simulink model "PMSM_DPCC_NLESO_MRAS"  (R2022a)
settings: Solver=FixedStepDiscrete  StartTime=0.0  StopTime=2  FixedStep=Ts  RelTol=1e-3
InitFcn:
  | Ts = 5e-7;%仿真步长
  | Tpwm = 1e-4;%开关周期
  | Tsample = Tpwm/1;%采样周期/控制周期
  | Tspeed = Tsample;%转速采样周期
  | Pn = 4;%电机极对数
  | Ls = 8.5e-3;%定子电感，采用隐极的，Ld=Lq=Ls
  | Rs = 3;%定子电阻
  | flux = 0.1688;%永磁体磁链
  | Vdc = 311;%直流母线电压
  | iqmax = 20;%额定电流
  | J = 5e-3;%转动惯量
  | B = 2.5e-3;%阻尼系数
  | n_init = 0;%初始转速
  | 
  | %这是DSP内部的控制器参数
  | Ls1 = 1*Ls;%电感参数设置为实际电感
  | Ld1 = Ls1;
  | Lq1 = Ls1;
  | Rs1 = 1*Rs;%电阻参数设置为实际电阻
  | flux1 =1*flux;%磁链参数设置为实际磁链
undefined symbols (not defined in the file): DiscIntNeverNeededParam, magnitude
libraries: simulink x9, slpidlib x2, spsDCVoltageSourceLib x1, spsPermanentMagnetSynchronousMachineLib x1, spsUniversalBridgeLib x1, spspowerguiLib x1
(part 2 of 2)

== matlab function PMSM_DPCC_NLESO_MRAS/SVPWM/电压采集模块 ==
  data: T1 input; udk output; T2 input; N input; uqk output; theta input; Tpwm input; Vdc input; wk input
function [udk,uqk] = fcn(T1,T2,N,theta,Tpwm,Vdc,wk)
%初始化
    Sa1 = 1;
    Sb1 = 1;
    Sc1 = 1;
    
    Sa2 = 1;
    Sb2 = 1;
    Sc2 = 1;
%%
%各个扇区对应的N分布为3 1 5 4 6 2 
%第I扇区的T1对应电压矢量100，T2对应电压矢量110；
%第II扇区的T1对应电压矢量010，T2对应电压矢量110；
%第III扇区的T1对应电压矢量010，T2对应电压矢量011；
%第IV扇区的T1对应电压矢量001，T2对应电压矢量011；
%第V扇区的T1对应电压矢量001，T2对应电压矢量101；
%第VI扇区的T1对应电压矢量100，T2对应电压矢量101；
%%
%翻译一下
%N=1的T1对应电压矢量010，T2对应电压矢量110；
%N=2的T1对应电压矢量100，T2对应电压矢量101；
%N=3的T1对应电压矢量100，T2对应电压矢量110；
%N=4的T1对应电压矢量001，T2对应电压矢量011；
%N=5的T1对应电压矢量010，T2对应电压矢量011；
%N=6的T1对应电压矢量001，T2对应电压矢量101；
%%
%相电压与开关函数的关系为：
%VaN = Vdc/3*(2*Sa-Sb-Sc);
%VbN = Vdc/3*(2*Sb-Sa-Sc);
%VcN = Vdc/3*(2*Sc-Sa-Sb);

if N==1
    Sa1 = 0;
    Sb1 = 1;
    Sc1 = 0;
    
    Sa2 = 1;
    Sb2 = 1;
    Sc2 = 0;
    
    
elseif N==2
    Sa1 = 1;
    Sb1 = 0;
    Sc1 = 0;
    
    Sa2 = 1;
    Sb2 = 0;
    Sc2 = 1;
    
    
 elseif N==3
    Sa1 = 1;
    Sb1 = 0;
    Sc1 = 0;
    
    Sa2 = 1;
    Sb2 = 1;
    Sc2 = 0;
    
    
 elseif N==4
    Sa1 = 0;
    Sb1 = 0;
    Sc1 = 1;
    
    Sa2 = 0;
    Sb2 = 1;
    Sc2 = 1;
    
    
 elseif N==5
    Sa1 = 0;
    Sb1 = 1;
    Sc1 = 0;
    
    Sa2 = 0;
    Sb2 = 1;
    Sc2 = 1;
    
    
 elseif N==6
    Sa1 = 0;
    Sb1 = 0;
    Sc1 = 1;
    
    Sa2 = 1;
    Sb2 = 0;
    Sc2 = 1;
end

VaN = Vdc/3*(2*Sa1-Sb1-Sc1)*T1/Tpwm+Vdc/3*(2*Sa2-Sb2-Sc2)*T2/Tpwm;
VbN = Vdc/3*(2*Sb1-Sa1-Sc1)*T1/Tpwm+Vdc/3*(2*Sb2-Sa2-Sc2)*T2/Tpwm;
VcN = Vdc/3*(2*Sc1-Sa1-Sb1)*T1/Tpwm+Vdc/3*(2*Sc2-Sa2-Sb2)*T2/Tpwm;

    
    if wk==0
        m = 1;
    else
        m = (2*sin(0.5*wk*Tpwm))/(wk*Tpwm);%平均值系数
    end
	theta_compen = theta+0.5*wk*Tpwm;
    trans = 2/3*m*[cos(theta_compen) cos(theta_compen-2*pi/3) cos(theta_compen+2*pi/3);
        -sin(theta_compen) -sin(theta_compen-2*pi/3) -sin(theta_compen+2*pi/3);];
    
VabcN =[VaN;VbN;VcN];
        %按顺序取出各开关状态，转化为列向量。上式是由开关状态与相电压的关系得到的。
        udqk = trans*VabcN;
        udk = udqk(1);
        uqk = udqk(2);
end

== matlab function PMSM_DPCC_NLESO_MRAS/RLS-based ==
  data: Mesk_1 input; Nesk_1 input; Mesk output; delta_udk_1 input; delta_idpk input; delta_idk input; delta_iqpk input; delta_iqk input; delta_uqk input; Tsample input; Ls input; iqmax input; lanbuda1 input; timecnt input; Nesk output
function [Mesk,Nesk]  = fcn(Mesk_1,Nesk_1,delta_udk_1,delta_idpk,delta_idk,delta_iqpk,delta_iqk,delta_uqk,Tsample,Ls,iqmax,lanbuda1,timecnt)
    Ts = Tsample;

    M = Ts/Ls;
    N=3;
    
    ref = 1.5;
    
    Hm = lanbuda1*(iqmax/M)^2*ref;
    Hn = lanbuda1*(iqmax/N)^2/4;
    
    %    Hn = 1e5;
    %end
% Mesk = M;
    if timecnt == 0.5 %&& timecnt <= 1.2
        Mesk = Ts/(0.6*Ls);
        Nesk = N*0.6;
    elseif timecnt == 1.2
        Mesk = Ts/(1.5*Ls);
        Nesk = N*1.5;
    else
        Mesk = Mesk_1-delta_udk_1*(delta_idpk-delta_idk)/Hm;%fix M
        Nesk = Nesk_1+(delta_iqpk-delta_iqk)*Mesk_1*delta_uqk/Hn;%fix R
    end

   
    

end
